simulink model "Concatenate"  (R2014a)
settings: Solver=ode45  StartTime=0.0  StopTime=10.0  RelTol=1e-3
libraries: hdlsllib x1
settings Model: Creator=Shiyu  LastModifiedBy=Shiyu

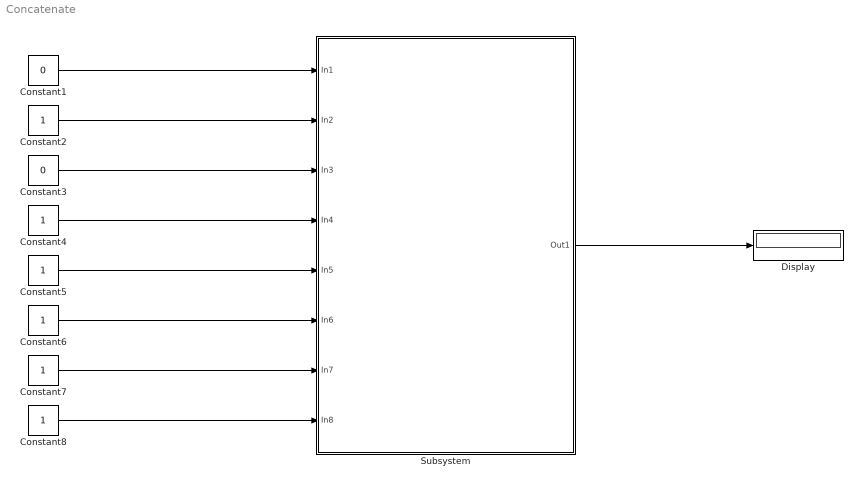
== system Concatenate ==
  Constant1 : Constant  Value=0  OutDataTypeStr=boolean
  Constant{2,4..8} (6 alike) : Constant  OutDataTypeStr=boolean
  Constant3 : Constant  Value=0  OutDataTypeStr=boolean
  Display : Display
  Subsystem : Subsystem
  wires:
  Constant1/1 -> Subsystem/1(In1)
  Constant2/1 -> Subsystem/2(In2)
  Constant3/1 -> Subsystem/3(In3)
  Constant4/1 -> Subsystem/4(In4)
  Constant5/1 -> Subsystem/5(In5)
  Constant6/1 -> Subsystem/6(In6)
  Constant7/1 -> Subsystem/7(In7)
  Constant8/1 -> Subsystem/8(In8)
  Subsystem/1(Out1) -> Display/1

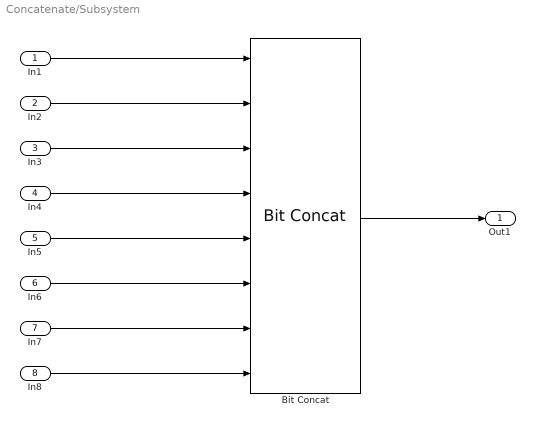
== system Concatenate/Subsystem ==
  In1 : Inport  OutDataTypeStr=boolean  SampleTime=1
  In2 : Inport  Port=2  OutDataTypeStr=boolean  SampleTime=1
  In3 : Inport  Port=3  OutDataTypeStr=boolean  SampleTime=1
  In4 : Inport  Port=4  OutDataTypeStr=boolean  SampleTime=1
  In5 : Inport  Port=5  OutDataTypeStr=boolean  SampleTime=1
  In6 : Inport  Port=6  OutDataTypeStr=boolean  SampleTime=1
  In7 : Inport  Port=7  OutDataTypeStr=boolean  SampleTime=1
  In8 : Inport  Port=8  OutDataTypeStr=boolean  SampleTime=1
  Bit Concat : hdlsllib/HDL Operations/Bit Concat  numInputs=8
  Out1 : Outport
  wires:
  In7/1 -> Bit Concat/7
  In4/1 -> Bit Concat/4
  Bit Concat/1 -> Out1/1
  In6/1 -> Bit Concat/6
  In5/1 -> Bit Concat/5
  In8/1 -> Bit Concat/8
  In1/1 -> Bit Concat/1
  In3/1 -> Bit Concat/3
  In2/1 -> Bit Concat/2
